simulink subsystem "SCIInAbstractionMotorSwap"  (R2024b)
settings: Solver=VariableStepAuto  StartTime=0.0  StopTime=10.0  RelTol=1e-3
values from neighbouring files (symbols this model uses):
  Ts = T_pwm    [mcbMotorSwapData.m]
undefined symbols (not defined in the file or in its folder): inverter
libraries: simulink x1, svdutilitieslib x1
settings Model: Creator=The MathWorks, Inc.  LastModifiedBy=snarayan
settings RTWCC: GPUComputeCapability=3.5

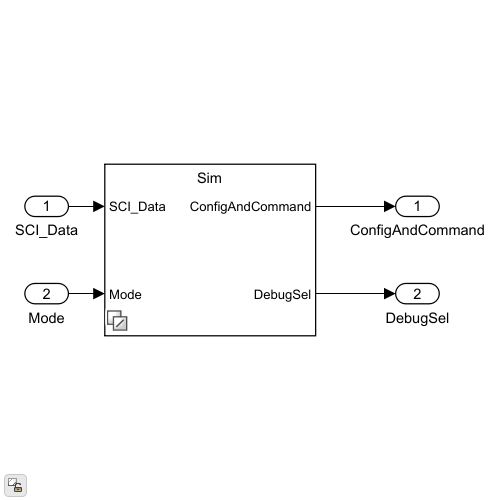
[thumbnail: Simulink's stored preview of the top-level diagram]
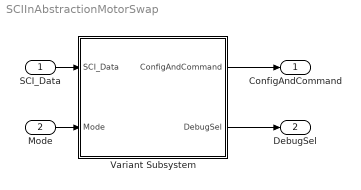
== system SCIInAbstractionMotorSwap ==
  SCI_Data : Inport
  Mode : Inport  Port=2
  Variant Subsystem : Subsystem  Variant=on  VariantControlMode=sim codegen switching
  ConfigAndCommand : Outport
  DebugSel : Outport  Port=2
  wires:
  SCI_Data/1 -> Variant Subsystem/1(SCI_Data)
  Variant Subsystem/2(DebugSel) -> DebugSel/1
  Variant Subsystem/1(ConfigAndCommand) -> ConfigAndCommand/1
  Mode/1 -> Variant Subsystem/2(Mode)

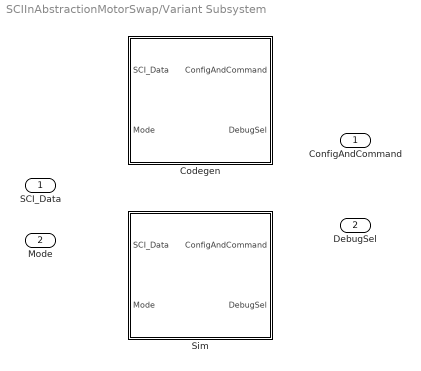
== system SCIInAbstractionMotorSwap/Variant Subsystem ==
  SCI_Data : Inport
  Mode : Inport  Port=2
  Codegen : Subsystem  VariantControl=(codegen)
  Sim : Subsystem  VariantControl=(sim)
  ConfigAndCommand : Outport
  DebugSel : Outport  Port=2

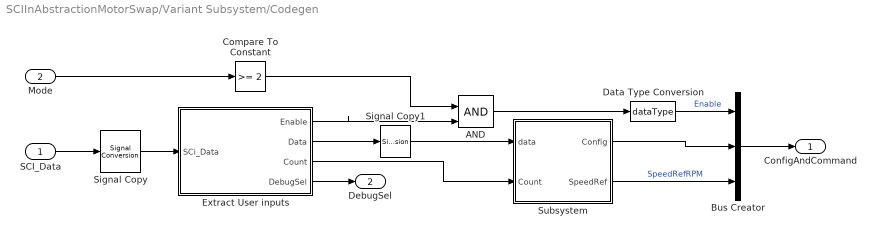
== system SCIInAbstractionMotorSwap/Variant Subsystem/Codegen ==
  SCI_Data : Inport
  Mode : Inport  Port=2
  AND : Logic  IconShape=distinctive  AllPortsSameDT=off  OutDataTypeStr=boolean
  Bus Creator : BusCreator  Inputs=3
  Compare To Constant : simulink/Logic and Bit Operations/Compare To Constant  relop=>=  const=2  OutDataTypeStr=boolean
  Data Type Conversion : DataTypeConversion  OutDataTypeStr=dataType  RndMeth=Simplest  SaturateOnIntegerOverflow=off
  Extract User inputs : Subsystem
  Signal Copy : SignalConversion  OverrideOpt=off
  Signal Copy1 : SignalConversion  OverrideOpt=on
  Subsystem : Subsystem
  ConfigAndCommand : Outport
  DebugSel : Outport  Port=2
  wires:
  Subsystem/2(SpeedRef) -> Bus Creator/3  "SpeedRefRPM"
  Signal Copy1/1 -> Subsystem/1(data)
  Signal Copy/1 -> Extract User inputs/1(SCi_Data)
  AND/1 -> Data Type Conversion/1
  Subsystem/1(Config) -> Bus Creator/2
  Extract User inputs/3(Count) -> Subsystem/2(Count)
  Extract User inputs/2(Data) -> Signal Copy1/1
  Extract User inputs/1(Enable) -> AND/2
  Compare To Constant/1 -> AND/1
  Mode/1 -> Compare To Constant/1
  Extract User inputs/4(DebugSel) -> DebugSel/1
  SCI_Data/1 -> Signal Copy/1
  Data Type Conversion/1 -> Bus Creator/1  "Enable"
  Bus Creator/1 -> ConfigAndCommand/1

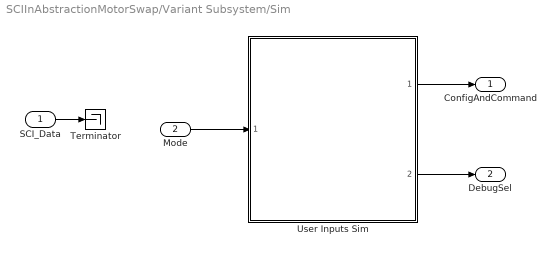
== system SCIInAbstractionMotorSwap/Variant Subsystem/Sim ==
  SCI_Data : Inport
  Mode : Inport  Port=2
  Terminator : Terminator
  User Inputs Sim : Subsystem  ReferencedSubsystem=SystemInputsSimMotorSwap
  ConfigAndCommand : Outport
  DebugSel : Outport  Port=2
  wires:
  User Inputs Sim/2 -> DebugSel/1
  User Inputs Sim/1 -> ConfigAndCommand/1
  Mode/1 -> User Inputs Sim/1
  SCI_Data/1 -> Terminator/1

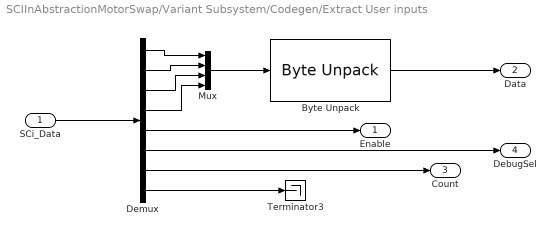
== system SCIInAbstractionMotorSwap/Variant Subsystem/Codegen/Extract User inputs ==
  SCi_Data : Inport
  Byte Unpack : svdutilitieslib/Byte Unpack  dimensions={[1]}  datatypes={'single'}  byteAlign=1  blockPlatform=tic2000
  Demux : Demux  Outputs=8
  Mux : Mux
  Terminator3 : Terminator
  Enable : Outport
  Data : Outport  Port=2
  Count : Outport  Port=3
  DebugSel : Outport  Port=4
  wires:
  Byte Unpack/1 -> Data/1
  Mux/1 -> Byte Unpack/1
  Demux/1 -> Mux/1
  Demux/2 -> Mux/2
  Demux/4 -> Mux/4
  Demux/3 -> Mux/3
  Demux/5 -> Enable/1
  Demux/6 -> DebugSel/1
  Demux/7 -> Count/1
  Demux/8 -> Terminator3/1
  SCi_Data/1 -> Demux/1

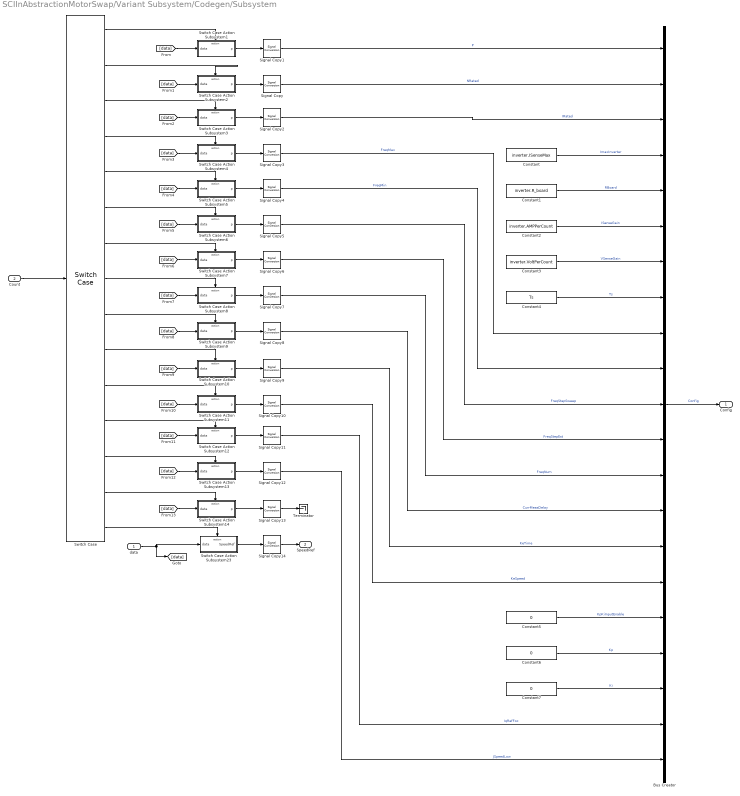
== system SCIInAbstractionMotorSwap/Variant Subsystem/Codegen/Subsystem ==
  data : Inport
  Count : Inport  Port=2
  Bus Creator : BusCreator  Inputs=21
  Constant : Constant  Value=inverter.ISenseMax  OutDataTypeStr=dataType
  Constant1 : Constant  Value=inverter.R_board  OutDataTypeStr=dataType
  Constant2 : Constant  Value=inverter.AMPPerCount  OutDataTypeStr=dataType
  Constant3 : Constant  Value=inverter.VoltPerCount  OutDataTypeStr=dataType
  Constant4 : Constant  Value=Ts  OutDataTypeStr=dataType
  Constant5 : Constant  Value=0  OutDataTypeStr=dataType
  Constant6 : Constant  Value=0  OutDataTypeStr=dataType
  Constant7 : Constant  Value=0  OutDataTypeStr=dataType
  Signal Copy{,1..14} (15 alike) : SignalConversion  OverrideOpt=on
  Switch Case : SwitchCase  CaseConditions={1 2 3 4 5 6 7 8 9 10 11 12 13 14 15}  ShowDefaultCase=off
  Switch Case Action Subsystem1 : Subsystem  TreatAsAtomicUnit=on
  Switch Case Action Subsystem10 : Subsystem  TreatAsAtomicUnit=on
  Switch Case Action Subsystem11 : Subsystem  TreatAsAtomicUnit=on
  Switch Case Action Subsystem12 : Subsystem  TreatAsAtomicUnit=on
  Switch Case Action Subsystem13 : Subsystem  TreatAsAtomicUnit=on
  Switch Case Action Subsystem14 : Subsystem  TreatAsAtomicUnit=on
  Switch Case Action Subsystem2 : Subsystem  TreatAsAtomicUnit=on
  Switch Case Action Subsystem23 : Subsystem  TreatAsAtomicUnit=on
  Switch Case Action Subsystem3 : Subsystem  TreatAsAtomicUnit=on
  Switch Case Action Subsystem4 : Subsystem  TreatAsAtomicUnit=on
  Switch Case Action Subsystem5 : Subsystem  TreatAsAtomicUnit=on
  Switch Case Action Subsystem6 : Subsystem  TreatAsAtomicUnit=on
  Switch Case Action Subsystem7 : Subsystem  TreatAsAtomicUnit=on
  Switch Case Action Subsystem8 : Subsystem  TreatAsAtomicUnit=on
  Switch Case Action Subsystem9 : Subsystem  TreatAsAtomicUnit=on
  Terminator : Terminator
  Config : Outport
  SpeedRef : Outport  Port=2
  wires:
  Signal Copy14/1 -> SpeedRef/1
  Signal Copy13/1 -> Terminator/1
  Signal Copy12/1 -> Bus Creator/21  "JSpeedLow"
  Signal Copy11/1 -> Bus Creator/20  "IqRefFoc"
  Constant7/1 -> Bus Creator/19  "Ki"
  Constant6/1 -> Bus Creator/18  "Kp"
  Constant5/1 -> Bus Creator/17  "KpKiInputEnable"
  Signal Copy10/1 -> Bus Creator/16  "KeSpeed"
  Signal Copy9/1 -> Bus Creator/15  "KeTime"
  Signal Copy8/1 -> Bus Creator/14  "CurrMeasDelay"
  Signal Copy7/1 -> Bus Creator/13  "FreqNum"
  Signal Copy6/1 -> Bus Creator/12  "FreqStepEst"
  Signal Copy5/1 -> Bus Creator/11  "FreqStepSweep"
  Signal Copy4/1 -> Bus Creator/10  "FreqMin"
  Signal Copy3/1 -> Bus Creator/9  "FreqMax"
  Constant4/1 -> Bus Creator/8  "Ts"
  Constant3/1 -> Bus Creator/7  "VSenseGain"
  Constant2/1 -> Bus Creator/6  "ISenseGain"
  Constant1/1 -> Bus Creator/5  "RBoard"
  Constant/1 -> Bus Creator/4  "ImaxInverter"
  Signal Copy2/1 -> Bus Creator/3  "IRated"
  Switch Case Action Subsystem14/1(p) -> Signal Copy13/1
  Switch Case Action Subsystem13/1(p) -> Signal Copy12/1
  Switch Case Action Subsystem12/1(p) -> Signal Copy11/1
  Switch Case Action Subsystem11/1(p) -> Signal Copy10/1
  Switch Case Action Subsystem10/1(p) -> Signal Copy9/1
  Switch Case Action Subsystem9/1(p) -> Signal Copy8/1
  Switch Case Action Subsystem8/1(p) -> Signal Copy7/1
  Switch Case Action Subsystem7/1(p) -> Signal Copy6/1
  Switch Case Action Subsystem6/1(p) -> Signal Copy5/1
  Switch Case Action Subsystem5/1(p) -> Signal Copy4/1
  Switch Case Action Subsystem4/1(p) -> Signal Copy3/1
  Switch Case Action Subsystem3/1(p) -> Signal Copy2/1
  [data] -> Switch Case Action Subsystem14/1(data)
  [data] -> Switch Case Action Subsystem13/1(data)
  [data] -> Switch Case Action Subsystem12/1(data)
  [data] -> Switch Case Action Subsystem11/1(data)
  [data] -> Switch Case Action Subsystem10/1(data)
  [data] -> Switch Case Action Subsystem9/1(data)
  [data] -> Switch Case Action Subsystem8/1(data)
  [data] -> Switch Case Action Subsystem7/1(data)
  Switch Case/14 -> Switch Case Action Subsystem14/Action
  Switch Case/13 -> Switch Case Action Subsystem13/Action
  Switch Case/12 -> Switch Case Action Subsystem12/Action
  Switch Case/11 -> Switch Case Action Subsystem11/Action
  Switch Case/10 -> Switch Case Action Subsystem10/Action
  Switch Case/9 -> Switch Case Action Subsystem9/Action
  Switch Case/8 -> Switch Case Action Subsystem8/Action
  Switch Case/7 -> Switch Case Action Subsystem7/Action
  [data] -> Switch Case Action Subsystem6/1(data)
  Switch Case/6 -> Switch Case Action Subsystem6/Action
  [data] -> Switch Case Action Subsystem5/1(data)
  Switch Case/5 -> Switch Case Action Subsystem5/Action
  [data] -> Switch Case Action Subsystem4/1(data)
  Switch Case/4 -> Switch Case Action Subsystem4/Action
  [data] -> Switch Case Action Subsystem3/1(data)
  Switch Case/3 -> Switch Case Action Subsystem3/Action
  [data] -> Switch Case Action Subsystem2/1(data)
  [data] -> Switch Case Action Subsystem1/1(data)
  Signal Copy1/1 -> Bus Creator/1  "P"
  Signal Copy/1 -> Bus Creator/2  "NRated"
  Switch Case Action Subsystem2/1(p) -> Signal Copy/1
  Switch Case/2 -> Switch Case Action Subsystem2/Action
  Switch Case Action Subsystem1/1(p) -> Signal Copy1/1
  Switch Case/1 -> Switch Case Action Subsystem1/Action
  Switch Case Action Subsystem23/1(SpeedRef) -> Signal Copy14/1
  data/1 -> Switch Case Action Subsystem23/1(data), [data]
  Switch Case/15 -> Switch Case Action Subsystem23/Action
  Count/1 -> Switch Case/1
  Bus Creator/1 -> Config/1  "Config"

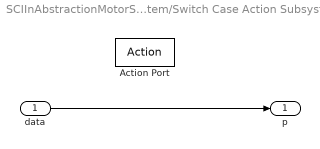
== system SCIInAbstractionMotorSwap/Variant Subsystem/Codegen/Subsystem/Switch Case Action Subsystem1 ==
  data : Inport
  Action Port : ActionPort
  p : Outport
  wires:
  data/1 -> p/1

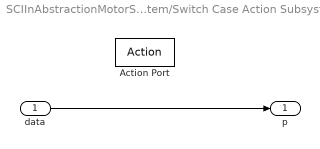
== system SCIInAbstractionMotorSwap/Variant Subsystem/Codegen/Subsystem/Switch Case Action Subsystem10 ==
  data : Inport
  Action Port : ActionPort
  p : Outport
  wires:
  data/1 -> p/1

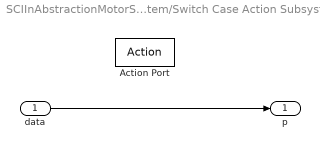
== system SCIInAbstractionMotorSwap/Variant Subsystem/Codegen/Subsystem/Switch Case Action Subsystem11 ==
  data : Inport
  Action Port : ActionPort
  p : Outport
  wires:
  data/1 -> p/1

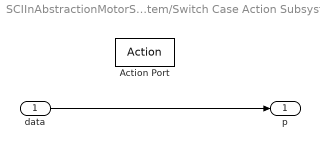
== system SCIInAbstractionMotorSwap/Variant Subsystem/Codegen/Subsystem/Switch Case Action Subsystem12 ==
  data : Inport
  Action Port : ActionPort
  p : Outport
  wires:
  data/1 -> p/1

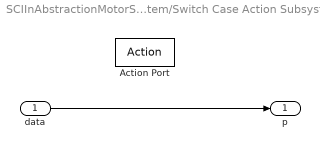
== system SCIInAbstractionMotorSwap/Variant Subsystem/Codegen/Subsystem/Switch Case Action Subsystem13 ==
  data : Inport
  Action Port : ActionPort
  p : Outport
  wires:
  data/1 -> p/1

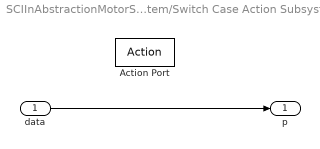
== system SCIInAbstractionMotorSwap/Variant Subsystem/Codegen/Subsystem/Switch Case Action Subsystem14 ==
  data : Inport
  Action Port : ActionPort
  p : Outport
  wires:
  data/1 -> p/1

== system SCIInAbstractionMotorSwap/Variant Subsystem/Codegen/Subsystem/Switch Case Action Subsystem2 ==
  data : Inport
  Action Port : ActionPort
  p : Outport
  wires:
  data/1 -> p/1

== system SCIInAbstractionMotorSwap/Variant Subsystem/Codegen/Subsystem/Switch Case Action Subsystem23 ==
  data : Inport
  Action Port : ActionPort
  SpeedRef : Outport
  wires:
  data/1 -> SpeedRef/1

== system SCIInAbstractionMotorSwap/Variant Subsystem/Codegen/Subsystem/Switch Case Action Subsystem3 ==
  data : Inport
  Action Port : ActionPort
  p : Outport
  wires:
  data/1 -> p/1

== system SCIInAbstractionMotorSwap/Variant Subsystem/Codegen/Subsystem/Switch Case Action Subsystem4 ==
  data : Inport
  Action Port : ActionPort
  p : Outport
  wires:
  data/1 -> p/1

== system SCIInAbstractionMotorSwap/Variant Subsystem/Codegen/Subsystem/Switch Case Action Subsystem5 ==
  data : Inport
  Action Port : ActionPort
  p : Outport
  wires:
  data/1 -> p/1

== system SCIInAbstractionMotorSwap/Variant Subsystem/Codegen/Subsystem/Switch Case Action Subsystem6 ==
  data : Inport
  Action Port : ActionPort
  p : Outport
  wires:
  data/1 -> p/1

== system SCIInAbstractionMotorSwap/Variant Subsystem/Codegen/Subsystem/Switch Case Action Subsystem7 ==
  data : Inport
  Action Port : ActionPort
  p : Outport
  wires:
  data/1 -> p/1

== system SCIInAbstractionMotorSwap/Variant Subsystem/Codegen/Subsystem/Switch Case Action Subsystem8 ==
  data : Inport
  Action Port : ActionPort
  p : Outport
  wires:
  data/1 -> p/1

== system SCIInAbstractionMotorSwap/Variant Subsystem/Codegen/Subsystem/Switch Case Action Subsystem9 ==
  data : Inport
  Action Port : ActionPort
  p : Outport
  wires:
  data/1 -> p/1
